simulink model "Motor_1"  (R2022a)
settings: Solver=FixedStepAuto  StartTime=0.0  StopTime=10.0  RelTol=1e-3  EnableMultiTasking=on
libraries: mbedblockslib x6, simulink x1
settings Model: ExtModeTrigDuration=10  Creator=Matlab  LastModifiedBy=Matlab
settings OptimizationCC: EnhancedBackFolding=on  PassReuseOutputArgsAs=Individual arguments  ZeroExternalMemoryAtStartup=off  ZeroInternalMemoryAtStartup=off  MaxStackSize=64  OptimizeBlockOrder=speed  DifferentSizesBufferReuse=on  OptimizationCustomize=off  EfficientTunableParamExpr=on
settings DebuggingCC: ParameterTunabilityLossMsg=error
settings HardwareCC: ProdBitPerPointer=32  ProdBitPerSizeT=32  ProdBitPerPtrDiffT=32  ProdLargestAtomicInteger=Long  ProdLargestAtomicFloat=Double  ProdWordSize=32  ProdLongLongMode=on  ProdHWDeviceType=ARM Compatible->ARM Cortex
settings SFSimCC: MATLABDynamicMemAlloc=off
settings RTWCC: SystemTargetFile=ert.tlc  HardwareBoard=STM32 Nucleo F411RE  TemplateMakefile=ert_default_tmf  Toolchain=GNU Tools for ARM Embedded Processors
settings CodeAppCC: ForceParamTrailComments=on  IgnoreCustomStorageClasses=off  OperatorAnnotations=on  SimulinkDataObjDesc=on  SFDataObjDesc=on  InsertBlockDesc=on
settings ERTTargetCC: SupportContinuousTime=on  ExtModeTransport=3  ExtModeStaticAlloc=on  ExtModeStaticAllocSize=2000  ExtModeMexFile=ext_xcp  ExtModeIntrfLevel=Level2 - Open

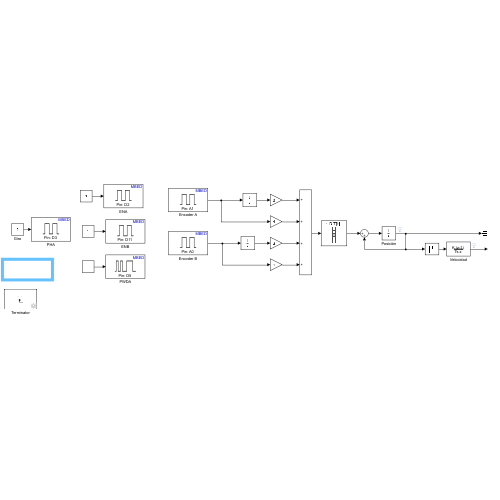
[thumbnail: Simulink's stored preview of the top-level diagram]
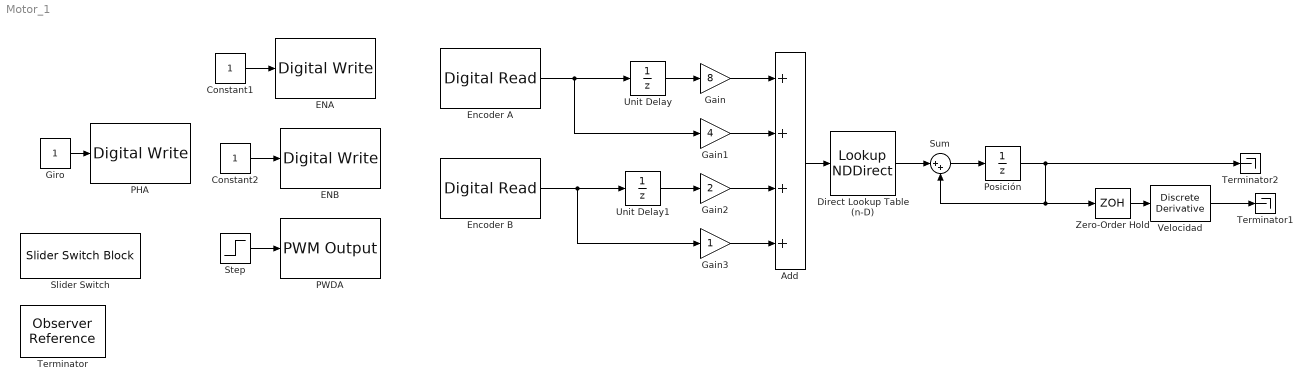
== system Motor_1 ==
  Add : Sum  Inputs=++++  OutDataTypeStr=double
  Constant1 : Constant
  Constant2 : Constant
  Direct Lookup Table (n-D) : LookupNDDirect  NumberOfTableDimensions=1  Table=[0,-1,1,0,1,0,0,-1,-1,0,0,1,0,1,-1,0]
  ENA : mbedblockslib/Digital Write  Pin=D2  Direction=output
      settings: SourceProductBaseCode=MICROBIT,NUCLEO,STMICRODIS
  ENB : mbedblockslib/Digital Write  Pin=D11  Direction=output
      settings: SourceProductBaseCode=MICROBIT,NUCLEO,STMICRODIS
  Encoder A : mbedblockslib/Digital Read  Pin=A1  Direction=input  SampleTime=0.0001
      settings: SourceProductBaseCode=MICROBIT,NUCLEO,STMICRODIS
  Encoder B : mbedblockslib/Digital Read  Pin=A0  Direction=input  SampleTime=0.0001
      settings: SourceProductBaseCode=MICROBIT,NUCLEO,STMICRODIS
  Gain : Gain  Gain=8
  Gain1 : Gain  Gain=4
  Gain2 : Gain  Gain=2
  Gain3 : Gain
  Giro : Constant
  PHA : mbedblockslib/Digital Write  Pin=D3  Direction=output
      settings: SourceProductBaseCode=MICROBIT,NUCLEO,STMICRODIS
  PWDA : mbedblockslib/PWM Output  Pin=D5  EnableInputFrequency=off  InitialFrequency=5000  InitialDutyCycle=0  NotificationType=None
      settings: SourceProductBaseCode=MICROBIT,NUCLEO,STMICRODIS
  Posición : UnitDelay  SampleTime=-1  HasFrameUpgradeWarning=on
  Slider Switch : SliderSwitchBlock
      settings: Values={{'Off', 'On'}, [0 1]}
  Step : Step  Time=0  After=50  SampleTime=0
  Sum : Sum  Inputs=|++
  Terminator : ObserverReference  ObserverModelName=untitled_Observer1
  Terminator1 : Terminator
  Terminator2 : Terminator
  Unit Delay : UnitDelay  SampleTime=-1  HasFrameUpgradeWarning=on
  Unit Delay1 : UnitDelay  SampleTime=-1  HasFrameUpgradeWarning=on
  Velocidad : simulink/Discrete/Discrete Derivative  gainval=1.0  ICPrevScaledInput=0.0  OutMin=[]  OutMax=[]  OutDataType=fixdt(1, 16)  OutScaling=2^-10  DoSatur=off
  Zero-Order Hold : ZeroOrderHold  SampleTime=0.01
  wires:
  Giro/1 -> PHA/1
  Constant1/1 -> ENA/1
  Constant2/1 -> ENB/1
  Step/1 -> PWDA/1
  Encoder B/1 -> Gain3/1, Unit Delay1/1
  Encoder A/1 -> Gain1/1, Unit Delay/1
  Unit Delay/1 -> Gain/1
  Unit Delay1/1 -> Gain2/1
  Gain/1 -> Add/1
  Gain1/1 -> Add/2
  Gain2/1 -> Add/3
  Gain3/1 -> Add/4
  Add/1 -> Direct Lookup Table (n-D)/1
  Direct Lookup Table (n-D)/1 -> Sum/1
  Sum/1 -> Posición/1
  Posición/1 -> Terminator2/1, Sum/2, Zero-Order Hold/1
  Zero-Order Hold/1 -> Velocidad/1
  Velocidad/1 -> Terminator1/1
